simulink model "njmsl"  (R2018a)
settings: Solver=VariableStepAuto  StartTime=0.0  StopTime=3  MaxStep=1e-3  RelTol=1e-3
undefined symbols (not defined in the file or in its folder): NJM
settings Model: Creator=Szalay  LastModifiedBy=Szalay

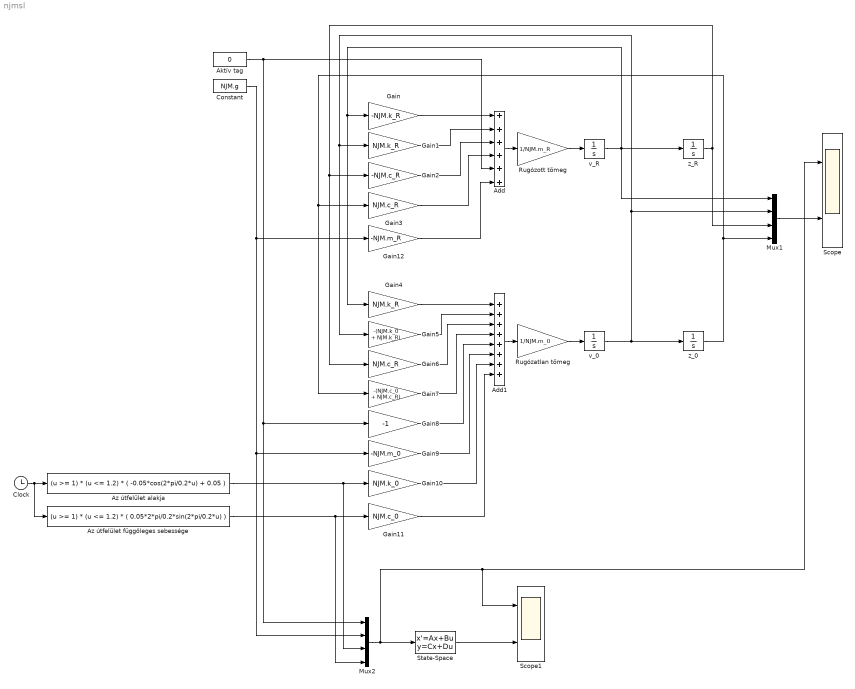
== system njmsl ==
  Add : Sum  Inputs=++++++
  Add1 : Sum  Inputs=++++++++
  Aktív tag : Constant  Value=0
  Az útfelület alakja : Fcn  Expr=(u >= 1) * (u <= 1.2) * ( -0.05*cos(2*pi/0.2*u) + 0.05 )
  Az útfelület függőleges sebessége : Fcn  Expr=(u >= 1) * (u <= 1.2) * ( 0.05*2*pi/0.2*sin(2*pi/0.2*u) )
  Clock : Clock
  Constant : Constant  Value=NJM.g
  Gain : Gain  Gain=-NJM.k_R
  Gain1 : Gain  Gain=NJM.k_R
  Gain10 : Gain  Gain=NJM.k_0
  Gain11 : Gain  Gain=NJM.c_0
  Gain12 : Gain  Gain=-NJM.m_R
  Gain2 : Gain  Gain=-NJM.c_R
  Gain3 : Gain  Gain=NJM.c_R
  Gain4 : Gain  Gain=NJM.k_R
  Gain5 : Gain  Gain=-(NJM.k_0 + NJM.k_R)
  Gain6 : Gain  Gain=NJM.c_R
  Gain7 : Gain  Gain=-(NJM.c_0 + NJM.c_R)
  Gain8 : Gain  Gain=-1
  Gain9 : Gain  Gain=-NJM.m_0
  Mux1 : Mux
  Mux2 : Mux
  Rugózatlan tömeg : Gain  Gain=1/NJM.m_0
  Rugózott tömeg : Gain  Gain=1/NJM.m_R
  Scope : Scope  NumInputPorts=2
  Scope1 : Scope  NumInputPorts=2
  State-Space : StateSpace  A=NJM.A  B=NJM.B  C=eye(4)  D=zeros(4)  InitialCondition=0
  v_0 : Integrator
  v_R : Integrator
  z_0 : Integrator
  z_R : Integrator
  wires:
  Rugózott tömeg/1 -> v_R/1
  Rugózatlan tömeg/1 -> v_0/1
  Add/1 -> Rugózott tömeg/1
  Gain/1 -> Add/1
  Gain1/1 -> Add/2
  Gain3/1 -> Add/4
  Gain2/1 -> Add/3
  Aktív tag/1 -> Add/5, Mux2/1, Gain8/1
  Constant/1 -> Gain12/1, Gain9/1, Mux2/2
  Gain6/1 -> Add1/3
  Gain7/1 -> Add1/4
  Gain5/1 -> Add1/2
  Gain4/1 -> Add1/1
  Add1/1 -> Rugózatlan tömeg/1
  Gain8/1 -> Add1/5
  Gain9/1 -> Add1/6
  Gain10/1 -> Add1/7
  Gain11/1 -> Add1/8
  v_R/1 -> Mux1/1, Gain4/1, Gain/1, z_R/1
  v_0/1 -> Mux1/2, Gain5/1, Gain1/1, z_0/1
  z_R/1 -> Mux1/3, Gain6/1, Gain2/1
  z_0/1 -> Mux1/4, Gain7/1, Gain3/1
  Mux1/1 -> Scope/2
  Az útfelület alakja/1 -> Mux2/3, Gain10/1
  State-Space/1 -> Scope1/2
  Gain12/1 -> Add/6
  Clock/1 -> Az útfelület alakja/1, Az útfelület függőleges sebessége/1
  Az útfelület függőleges sebessége/1 -> Mux2/4, Gain11/1
  Mux2/1 -> Scope1/1, Scope/1, State-Space/1
